simulink model "TeamA_PAsqualo_R19b"  (R2019b)
settings: Solver=VariableStepAuto  StartTime=0.0  StopTime=stop_time  FixedStep=0.05  RelTol=1e-3
InitFcn:
  | main_init
values from neighbouring files (symbols this model uses):
  a1 = rho * D^4 * alpha1    (= 0.000388302366464)    [data_current.m]    (also in main_init.m)
  a2 = -rho * D^3 * alpha2 * (1 - omega)    (= 0.0037030698432)    [data_current.m]    (also in main_init.m)
  ag = [Ax Ay Az]'    [init_modello.m]
  alpha1 = 0.0113    [data_current.m]    (also in main_init.m)
  alpha2 = -0.0091    [data_current.m]    (also in main_init.m)
  areaOfInterestCorner = [42.317744;10.915136; 0]    [init_controllo.m]    (also in missionA.m = [42.317744)
  bg = [Bx By Bz]'    [init_modello.m]
  cd_pitch = 0.7    [init_modello.m]
  cd_roll = 0.04    [init_modello.m]
  cd_x = 0.4    [init_modello.m]
  cd_y = 1    [init_modello.m]
  cd_yaw = 0.7    [init_modello.m]
  cd_z = 1    [init_modello.m]
  cg = [Cx Cy Cz]'    [init_modello.m]
  D = 0.076    [data_current.m]    (also in main_init.m)
  dead_zone_limit = 31.5    [data_current.m]    (also in main_init.m)
  dg = [Dx Dy Dz]'    [init_modello.m]
  eg = [Ex Ey Ez]'    [init_modello.m]
  fg = [Fx Fy Fz]'    [init_modello.m]
  g = 9.81    [init_modello.m]
  galleggiamento = 66.5386    [init_controllo.m]
  gg = [Gx Gy Gz]'    [init_modello.m]
  H0 = 0    [init_modello.m]
  init_position = [pointP(1),pointP(2),0.15,0,0,deg2rad(angle)]'    [appunti.m]    (also in init_modello.m = [pointP(1),pointP(2),0.15,0,0,deg2rad(alpha)]')
  init_velocity = [0 0 0 0 0 0]'    [init_modello.m]
  initial_state_cov = blkdiag(diag(cov_gps(1,1:2)), cov_depth*eye(n_state_filter-2))    [init_navigazione.m]
  Ixx = 0.93304097392    [init_modello.m]
  Ixy = 0    [init_modello.m]
  Ixz = 0    [init_modello.m]
  Iyy = 25.58745481378    (= 25.5874548138)    [init_modello.m]
  Iyz = 0    [init_modello.m]
  Izz = 25.58745481378    (= 25.5874548138)    [init_modello.m]
  K_i_heave_div = 20    [init_controllo.m]
  K_i_heave_pos = 1    [init_controllo.m]
  K_i_heave_surf = 20    [init_controllo.m]
  K_i_heave_trans = 5    [init_controllo.m]
  K_i_heave_turn = 5    [init_controllo.m]
  K_i_pitch_div = 0    [init_controllo.m]
  K_i_pitch_pos = 0.1*0    (= 0)    [init_controllo.m]
  K_i_pitch_surf = 0    [init_controllo.m]
  K_i_pitch_trans = 0    [init_controllo.m]
  K_i_pitch_turn = 0    [init_controllo.m]
  K_i_roll_div = 0    [init_controllo.m]
  K_i_roll_pos = 0.1*0    (= 0)    [init_controllo.m]
  K_i_roll_surf = 1    [init_controllo.m]
  K_i_roll_trans = 0    [init_controllo.m]
  K_i_roll_turn = 0    [init_controllo.m]
  K_i_surge_div = 3    [init_controllo.m]
  K_i_surge_pos = 0.1679*30    (= 5.037)    [init_controllo.m]
  K_i_surge_surf = 3    [init_controllo.m]
  K_i_surge_trans = 0.1679*15    (= 2.5185)    [init_controllo.m]
  K_i_surge_turn = 0.1679*60    (= 10.074)    [init_controllo.m]
  K_i_sway_div = 6    [init_controllo.m]
  K_i_sway_pos = 5    [init_controllo.m]
  K_i_sway_surf = 3    [init_controllo.m]
  K_i_sway_trans = 2    [init_controllo.m]
  K_i_sway_turn = 50    [init_controllo.m]
  K_i_yaw_div = 0    [init_controllo.m]
  K_i_yaw_pos = 1    [init_controllo.m]
  K_i_yaw_surf = 0    [init_controllo.m]
  K_i_yaw_trans = 20    [init_controllo.m]
  K_p_heave_div = 200    [init_controllo.m]
  K_p_heave_pos = 320    [init_controllo.m]
  K_p_heave_surf = 200    [init_controllo.m]
  K_p_heave_trans = 170    [init_controllo.m]
  K_p_heave_turn = 170    [init_controllo.m]
  K_p_phi_div = 0.15    [init_controllo.m]
  K_p_phi_pos = 1*0.1    (= 0.1)    [init_controllo.m]
  K_p_phi_surf = 0.15    [init_controllo.m]
  K_p_phi_trans = 0.1    [init_controllo.m]
  K_p_phi_turn = 0.1    [init_controllo.m]
  K_p_pitch_div = 50    [init_controllo.m]
  K_p_pitch_pos = 25    [init_controllo.m]
  K_p_pitch_surf = 50    [init_controllo.m]
  K_p_pitch_trans = 25    [init_controllo.m]
  K_p_pitch_turn = 25    [init_controllo.m]
  K_p_psi_div = 0.3    [init_controllo.m]
  K_p_psi_pos = 0.25    [init_controllo.m]
  K_p_psi_surf = 0.3    [init_controllo.m]
  K_p_psi_trans = 0.2    [init_controllo.m]
  K_p_roll_div = 10    [init_controllo.m]
  K_p_roll_pos = 0.1*40    (= 4)    [init_controllo.m]
  K_p_roll_surf = 10    [init_controllo.m]
  K_p_roll_trans = 0.1*40    (= 4)    [init_controllo.m]
  K_p_roll_turn = 4    [init_controllo.m]
  K_p_surge_div = 80    [init_controllo.m]
  K_p_surge_pos = 13.7782*2.5    (= 34.4455)    [init_controllo.m]
  K_p_surge_surf = 80    [init_controllo.m]
  K_p_surge_trans = 20    [init_controllo.m]
  K_p_surge_turn = 150    [init_controllo.m]
  K_p_sway_div = 100    [init_controllo.m]
  K_p_sway_pos = 90    [init_controllo.m]
  K_p_sway_surf = 80    [init_controllo.m]
  K_p_sway_trans = 80    [init_controllo.m]
  K_p_sway_turn = 200    [init_controllo.m]
  K_p_th_div = 0.3    [init_controllo.m]
  K_p_th_pos = 0.1    [init_controllo.m]
  K_p_th_surf = 0.3    [init_controllo.m]
  K_p_th_trans = 0.1    [init_controllo.m]
  K_p_th_turn = 0.1    [init_controllo.m]
  K_p_x_div = 0.12    [init_controllo.m]
  K_p_x_pos = 0.12    [init_controllo.m]
  K_p_x_surf = 0.12    [init_controllo.m]
  K_p_y_div = 0.6    [init_controllo.m]
  K_p_y_pos = 0.34    [init_controllo.m]
  K_p_y_surf = 0.1    [init_controllo.m]
  K_p_y_trans = 0.3    [init_controllo.m]
  K_p_y_turn = 0.3    [init_controllo.m]
  K_p_yaw_div = 70    [init_controllo.m]
  K_p_yaw_pos = 20    [init_controllo.m]
  K_p_yaw_surf = 70    [init_controllo.m]
  K_p_yaw_trans = 160    [init_controllo.m]
  K_p_z_div = 0.35    [init_controllo.m]
  K_p_z_pos = 0.2    [init_controllo.m]
  K_p_z_surf = 0.35    [init_controllo.m]
  K_p_z_trans = 0.10    (= 0.1)    [init_controllo.m]
  K_p_z_turn = 0.1    [init_controllo.m]
  Kadd = 0    [init_modello.m]
  m = 100    [init_modello.m]    (also in retta.m = p2-p1)
  Madd = -((((1/5)*(b^2-a^2)^2))*(alpha_0-beta_0))/((((2*(b^2-a^2)^2))+(b^2-a^2)^2)*(alpha_0-beta_0)*m)    [init_modello.m]
  ... (+59 more)
undefined symbols (not defined in the file or in its folder): DiscIntNeverNeededParam, initial_state
libraries: simulink x2, vrlib x1
(part 5 of 6)

== matlab function TeamA_PAsqualo_R19b/controller1/diving controller/heave_controller/Heave PID controller/compute_position_errors ==
  settings: updateMethod=DISCRETE  sampleTime=0.1
  data: enable input size=1; err_pos output size=1; ref input size=[12 1]; est_state input size=[12 1]; w_des output size=1; areaOfInterestCorner parameter
function [err_pos, w_des] = fcn(enable, ref, est_state,areaOfInterestCorner)
references_NED = zeros(3,1);
est_state_NED  = zeros(3,1);
phi = est_state(4);
th  = est_state(5);
psi = est_state(6);
coder.extrinsic('evalin','wgs84Ellipsoid','geodetic2ned');
orig = [areaOfInterestCorner(1)   areaOfInterestCorner(2)   areaOfInterestCorner(3)]'; %origine terna NED
wgs84 = wgs84Ellipsoid;
err_pos = 0;
w_des = 0;
if enable == 1
    % Cambiamento di riferimento da WGS84 a NED frame
   [x_ref, y_ref, z_ref] = geodetic2ned(ref(1),ref(2),ref(3),orig(1),orig(2),orig(3),wgs84);
   references_NED = [x_ref, y_ref, z_ref]';
   [x_est, y_est, z_est] = geodetic2ned(est_state(1),est_state(2),est_state(3),orig(1),orig(2),orig(3),wgs84);
   est_state_NED  =  [x_est, y_est, z_est]';
   est_state_NED = [est_state_NED(1);est_state_NED(2);est_state(3)];
   % Calcolo errore posizione da NED a BODY frame
   err_NED  = references_NED - est_state_NED;
   R_z_psi = [cos(psi)    sin(psi)     0;
              -sin(psi)   cos(psi)     0;
                 0           0         1];
          
   R_y_th =  [cos(th)        0      -sin(th);
                 0           1         0;
              sin(th)        0       cos(th)];
       
   R_x_phi = [   1           0             0;
                 0         cos(phi)    sin(phi);
                 0        -sin(phi)    cos(phi)];
          
   R_NB = ((R_z_psi')*(R_y_th')*(R_x_phi'))';
   err_pos_BODY = R_NB * err_NED;
   offset = 0.5;  % metri di distanza dal punto desiderato
   if err_pos_BODY(3) > offset
       err_pos = 0;
       w_des   = ref(9);
   end
   if err_pos_BODY(3) <= offset
       err_pos = err_pos_BODY(3);
       w_des   = 0;
   end
else
   err_pos = 0;
   w_des   = 0;
end
end

== matlab function TeamA_PAsqualo_R19b/controller1/diving controller/heave_controller/Heave PID controller/compute_velocity_error ==
  settings: updateMethod=DISCRETE  sampleTime=0.1
  data: enable input size=1; err_vel output size=1; v_des input size=1; est_meas input size=[12 1]
function err_vel = fcn(enable,v_des,est_meas)
if enable == 1
   err_vel =  v_des - est_meas(9);
else
    err_vel = 0;
end
end

== matlab function TeamA_PAsqualo_R19b/controller1/diving controller/pitch_controller/Pitch PID controller/compute_orientation_errors ==
  settings: updateMethod=DISCRETE  sampleTime=0.1
  data: enable input size=1; err_orient output size=1; ref input size=[12 1]; est_state input size=[12 1]
function err_orient = fcn(enable, ref, est_state)
coder.extrinsic('wrapToPi');
err_orient = 0;
phi = est_state(4);
th  = est_state(5);
%
J_inv = [1       0          -sin(th); 
         0   cos(phi)  cos(th)*sin(phi);
         0  -sin(phi)  cos(th)*cos(phi)];
if enable == 1
   err_orient_1 = wrapToPi(J_inv*([ref(4);ref(5);ref(6)] -...
                           [est_state(4);est_state(5);est_state(6)]));
else 
   err_orient_1 = zeros(3,1);
end
err_orient = err_orient_1(2);
end

== matlab function TeamA_PAsqualo_R19b/controller1/diving controller/pitch_controller/Pitch PID controller/compute_velocity_error ==
  settings: updateMethod=DISCRETE  sampleTime=0.1
  data: enable input size=1; err_vel output size=1; v_des input size=1; est_meas input size=[12 1]
function err_vel = fcn(enable,v_des,est_meas)
if enable == 1
   err_vel =  v_des - est_meas(11);
else
    err_vel = 0;
end
end

== matlab function TeamA_PAsqualo_R19b/controller1/diving controller/roll_controller/Roll PID controller/compute_orientation_errors ==
  settings: updateMethod=DISCRETE  sampleTime=0.1
  data: enable input size=1; err_orient output size=1; ref input size=[12 1]; est_state input size=[12 1]
function err_orient = fcn(enable, ref, est_state)
coder.extrinsic('wrapToPi');
err_orient = 0;
phi = est_state(4);
th  = est_state(5);
%
J_inv = [1       0          -sin(th); 
         0   cos(phi)  cos(th)*sin(phi);
         0  -sin(phi)  cos(th)*cos(phi)];
if enable == 1
   err_orient_1 = wrapToPi(J_inv*([ref(4);ref(5);ref(6)] -...
                           [est_state(4);est_state(5);est_state(6)]));
else 
   err_orient_1 = zeros(3,1);
end
err_orient = err_orient_1(1);
end

== matlab function TeamA_PAsqualo_R19b/controller1/diving controller/roll_controller/Roll PID controller/compute_velocity_error ==
  settings: updateMethod=DISCRETE  sampleTime=0.1
  data: enable input size=1; err_vel output size=1; v_des input size=1; est_meas input size=[12 1]
function err_vel = fcn(enable,v_des,est_meas)
if enable == 1
   err_vel =  v_des - est_meas(10);
else
    err_vel = 0;
end
end

== matlab function TeamA_PAsqualo_R19b/controller1/diving controller/surge_controller/Surge PID controller/compute_position_errors ==
  settings: updateMethod=DISCRETE  sampleTime=0.1
  data: enable input size=1; err_pos output size=1; ref input size=[12 1]; est_state input size=[12 1]; areaOfInterestCorner parameter
function err_pos = fcn(enable, ref, est_state,areaOfInterestCorner)
references_NED = zeros(3,1);
est_state_NED  = zeros(3,1);
phi = est_state(4);
th  = est_state(5);
psi = est_state(6);
coder.extrinsic('evalin','wgs84Ellipsoid','geodetic2ned');
orig = [areaOfInterestCorner(1)   areaOfInterestCorner(2)   areaOfInterestCorner(3)]'; %origine terna NED
wgs84 = wgs84Ellipsoid;
if enable == 1
    % Cambiamento di riferimento da WGS84 a NED frame
   [x_ref, y_ref, z_ref] = geodetic2ned(ref(1),ref(2),ref(3),orig(1),orig(2),orig(3),wgs84);
   references_NED = [x_ref, y_ref, z_ref]';
   [x_est, y_est, z_est] = geodetic2ned(est_state(1),est_state(2),est_state(3),orig(1),orig(2),orig(3),wgs84);
   est_state_NED  =  [x_est, y_est, est_state(3)]';
   % Calcolo errore posizione da NED a BODY frame
   err_NED  = references_NED - est_state_NED;
   R_z_psi = [cos(psi)    sin(psi)     0;
              -sin(psi)   cos(psi)     0;
                 0           0         1];
          
   R_y_th =  [cos(th)        0      -sin(th);
                 0           1         0;
              sin(th)        0       cos(th)];
       
   R_x_phi = [   1           0             0;
                 0         cos(phi)    sin(phi);
                 0        -sin(phi)    cos(phi)];
          
   R_NB = ((R_z_psi')*(R_y_th')*(R_x_phi'))';
   err_pos_BODY = R_NB * err_NED;

   err_pos = err_pos_BODY(1);
else
   err_pos = 0;
end
end

== matlab function TeamA_PAsqualo_R19b/controller1/diving controller/surge_controller/Surge PID controller/compute_velocity_error ==
  settings: updateMethod=DISCRETE  sampleTime=0.1
  data: enable input size=1; err_vel output size=1; v_des input size=1; est_meas input size=[12 1]
function err_vel = fcn(enable,v_des,est_meas)
if enable == 1
   err_vel =  v_des - est_meas(7);
else
    err_vel = 0;
end
end

== matlab function TeamA_PAsqualo_R19b/controller1/diving controller/sway_controller/Sway PID controller/compute_position_errors ==
  settings: updateMethod=DISCRETE  sampleTime=0.1
  data: enable input size=1; err_pos output size=1; ref input size=[12 1]; est_state input size=[12 1]; areaOfInterestCorner parameter
function err_pos = fcn(enable, ref, est_state,areaOfInterestCorner)
references_NED = zeros(3,1);
est_state_NED  = zeros(3,1);
phi = est_state(4);
th  = est_state(5);
psi = est_state(6);
coder.extrinsic('evalin','wgs84Ellipsoid','geodetic2ned');
orig = [areaOfInterestCorner(1)   areaOfInterestCorner(2)   areaOfInterestCorner(3)]'; %origine terna NED
wgs84 = wgs84Ellipsoid;
if enable == 1
    % Cambiamento di riferimento da WGS84 a NED frame
   [x_ref, y_ref, z_ref] = geodetic2ned(ref(1),ref(2),ref(3),orig(1),orig(2),orig(3),wgs84);
   references_NED = [x_ref, y_ref, z_ref]';
   [x_est, y_est, z_est] = geodetic2ned(est_state(1),est_state(2),est_state(3),orig(1),orig(2),orig(3),wgs84);
   est_state_NED  = [x_est, y_est, est_state(3)]';
   % Calcolo errore posizione da NED a BODY frame
   err_NED  = references_NED - est_state_NED;
   R_z_psi = [cos(psi)    sin(psi)     0;
              -sin(psi)   cos(psi)     0;
                 0           0         1];
          
   R_y_th =  [cos(th)        0      -sin(th);
                 0           1         0;
              sin(th)        0       cos(th)];
       
   R_x_phi = [   1           0             0;
                 0         cos(phi)    sin(phi);
                 0        -sin(phi)    cos(phi)];
          
   R_NB = ((R_z_psi')*(R_y_th')*(R_x_phi'))';
   err_pos_BODY = R_NB * err_NED;
   err_pos = err_pos_BODY(2);
else
   err_pos = 0;
end
end

== matlab function TeamA_PAsqualo_R19b/controller1/diving controller/sway_controller/Sway PID controller/compute_velocity_error ==
  settings: updateMethod=DISCRETE  sampleTime=0.1
  data: enable input size=1; err_vel output size=1; v_des input size=1; est_meas input size=[12 1]
function err_vel = fcn(enable,v_des,est_meas)
if enable == 1
   err_vel =  v_des - est_meas(8);
else
    err_vel = 0;
end
end

== matlab function TeamA_PAsqualo_R19b/controller1/diving controller/yaw_controller/Yaw PID controller/compute_orientation_errors ==
  settings: updateMethod=DISCRETE  sampleTime=0.1
  data: enable input size=1; err_orient output size=1; ref input size=[12 1]; est_state input size=[12 1]
function err_orient = fcn(enable, ref, est_state)
coder.extrinsic('wrapToPi');
err_orient = 0;
phi = est_state(4);
th  = est_state(5);
%
J_inv = [1       0          -sin(th); 
         0   cos(phi)  cos(th)*sin(phi);
         0  -sin(phi)  cos(th)*cos(phi)];
if enable == 1
   err_orient_1 = wrapToPi(J_inv*([ref(4);ref(5);ref(6)] -...
                           [est_state(4);est_state(5);est_state(6)]));
else 
   err_orient_1 = zeros(3,1);
end
err_orient = err_orient_1(3);
end

== matlab function TeamA_PAsqualo_R19b/controller1/diving controller/yaw_controller/Yaw PID controller/compute_velocity_error ==
  data: enable input; err_vel output; v_des input; est_meas input
function err_vel = fcn(enable,v_des,est_meas)
if enable == 1
   err_vel =  v_des - est_meas(12);
else
    err_vel = 0;
end

== matlab function TeamA_PAsqualo_R19b/controller1/positioning controller/heave_controller/Heave PID controller/compute_position_errors ==
  data: enable input; err_pos output; ref input; est_state input; areaOfInterestCorner parameter
function err_pos = fcn(enable, ref, est_state,areaOfInterestCorner)
references_NED = zeros(3,1);
est_state_NED  = zeros(3,1);
phi = est_state(4);
th  = est_state(5);
psi = est_state(6);
coder.extrinsic('evalin','wgs84Ellipsoid','geodetic2ned');   
orig = [areaOfInterestCorner(1)   areaOfInterestCorner(2)   areaOfInterestCorner(3)]'; %origine terna NED
wgs84 = wgs84Ellipsoid;
if enable == 1
    % Cambiamento di riferimento da WGS84 a NED frame
   [x_ref, y_ref, z_ref] = geodetic2ned(ref(1),ref(2),ref(3),orig(1),orig(2),orig(3),wgs84);
   references_NED = [x_ref, y_ref, z_ref]';
   [x_est, y_est, z_est] = geodetic2ned(est_state(1),est_state(2),est_state(3),orig(1),orig(2),orig(3),wgs84);
   est_state_NED  =  [x_est, y_est, est_state(3)]';
   % Calcolo errore posizione da NED a BODY frame
   err_NED  = references_NED - est_state_NED;
   R_z_psi = [cos(psi)    sin(psi)     0;
              -sin(psi)   cos(psi)     0;
                 0           0         1];
          
   R_y_th =  [cos(th)        0      -sin(th);
                 0           1         0;
              sin(th)        0       cos(th)];
       
   R_x_phi = [   1           0             0;
                 0         cos(phi)    sin(phi);
                 0        -sin(phi)    cos(phi)];
          
   R_NB = ((R_z_psi')*(R_y_th')*(R_x_phi'))';
   err_pos_BODY = R_NB * err_NED;
   err_pos = err_pos_BODY(3);
else
   err_pos = 0;
end
end

== matlab function TeamA_PAsqualo_R19b/controller1/positioning controller/heave_controller/Heave PID controller/compute_velocity_error ==
  data: enable input; err_vel output; v_des input; est_meas input
function err_vel = fcn(enable,v_des,est_meas)
err_vel = 0;
if enable == 1
   err_vel =  v_des - est_meas(9);
else 
    err_vel = 0;
end
end

== matlab function TeamA_PAsqualo_R19b/controller1/positioning controller/pitch_controller/Pitch PID controller/compute_orientation_errors ==
  data: enable input; err_orient output; ref input; est_state input
function err_orient = fcn(enable, ref, est_state)
coder.extrinsic('wrapToPi');
err_orient = 0;
phi = est_state(4);
th  = est_state(5);
%
J_inv = [1       0          -sin(th); 
         0   cos(phi)  cos(th)*sin(phi);
         0  -sin(phi)  cos(th)*cos(phi)];
if enable == 1
   err_orient_1 = wrapToPi(J_inv*([ref(4);ref(5);ref(6)] -...
                                [est_state(4);est_state(5);est_state(6)]));
else 
   err_orient_1 = zeros(3,1);
end
err_orient = err_orient_1(2);
end

== matlab function TeamA_PAsqualo_R19b/controller1/positioning controller/pitch_controller/Pitch PID controller/compute_velocity_error ==
  data: enable input; err_vel output; v_des input; est_meas input
function err_vel = fcn(enable,v_des,est_meas)
if enable == 1
   err_vel =  v_des - est_meas(11);
else
    err_vel = 0;
end
end

== matlab function TeamA_PAsqualo_R19b/controller1/positioning controller/roll_controller/Roll PID controller/compute_orientation_errors ==
  data: enable input; err_orient output; ref input; est_state input
function err_orient = fcn(enable, ref, est_state)
coder.extrinsic('wrapToPi');
err_orient = 0;
phi = est_state(4);
th  = est_state(5);
%
J_inv = [1       0          -sin(th); 
         0   cos(phi)  cos(th)*sin(phi);
         0  -sin(phi)  cos(th)*cos(phi)];
if enable == 1
   err_orient_1 = wrapToPi(J_inv*([ref(4);ref(5);ref(6)] -...
                           [est_state(4);est_state(5);est_state(6)]));
else 
   err_orient_1 = zeros(3,1);
end
err_orient = err_orient_1(1);
end

== matlab function TeamA_PAsqualo_R19b/controller1/positioning controller/roll_controller/Roll PID controller/compute_velocity_error ==
  data: enable input; err_vel output; v_des input; est_meas input
function err_vel = fcn(enable,v_des,est_meas)
if enable == 1
   err_vel =  v_des - est_meas(10);
else 
    err_vel = 0;
end
end

== matlab function TeamA_PAsqualo_R19b/controller1/positioning controller/surge_controller/Surge PID controller/compute_position_errors ==
  data: enable input; err_pos output; ref input; est_state input; u_des output; areaOfInterestCorner parameter
function [err_pos, u_des] = fcn(enable, ref, est_state,areaOfInterestCorner)
references_NED = zeros(3,1);
est_state_NED  = zeros(3,1);
phi = est_state(4);
th  = est_state(5);
psi = est_state(6);
coder.extrinsic('evalin','wgs84Ellipsoid','geodetic2ned');
orig = [areaOfInterestCorner(1)   areaOfInterestCorner(2)   areaOfInterestCorner(3)]'; %origine terna NED
wgs84 = wgs84Ellipsoid;
err_pos = 0;
u_des = 0;

if enable == 1
    % Cambiamento di riferimento da WGS84 a NED frame
   [x_ref, y_ref, z_ref] = geodetic2ned(ref(1),ref(2),ref(3),orig(1),orig(2),orig(3),wgs84);
   references_NED = [x_ref, y_ref, z_ref]';
   [x_est, y_est, z_est] = geodetic2ned(est_state(1),est_state(2),est_state(3),orig(1),orig(2),orig(3),wgs84);
   est_state_NED  =  [x_est, y_est, z_est]';
   est_state_NED = [est_state_NED(1);est_state_NED(2);est_state(3)];
   % Calcolo errore posizione da NED a BODY frame
   err_NED  = references_NED - est_state_NED;
   R_z_psi = [cos(psi)    sin(psi)     0;
              -sin(psi)   cos(psi)     0;
                 0           0         1];
          
   R_y_th =  [cos(th)        0      -sin(th);
                 0           1         0;
              sin(th)        0       cos(th)];
       
   R_x_phi = [   1           0             0;
                 0         cos(phi)    sin(phi);
                 0        -sin(phi)    cos(phi)];
          
   R_NB = ((R_z_psi')*(R_y_th')*(R_x_phi'))';
   err_pos_BODY = R_NB * err_NED;
   offset = 5;  % metri di distanza dal punto desiderato
   if abs(err_pos_BODY(1)) > offset
       err_pos = 0;
       u_des   = ref(7);
   end
   if abs(err_pos_BODY(1)) <= offset
       err_pos = err_pos_BODY(1);
       u_des   = 0;
   end
else
   err_pos = 0;
   u_des   = 0;
end
end

== matlab function TeamA_PAsqualo_R19b/controller1/positioning controller/surge_controller/Surge PID controller/compute_velocity_error ==
  data: enable input; err_vel output; v_des input; est_meas input
function err_vel = fcn(enable,v_des,est_meas)
if enable == 1
   err_vel =  v_des - est_meas(7);
else
    err_vel = 0;
end
end

== matlab function TeamA_PAsqualo_R19b/controller1/positioning controller/sway_controller/Sway PID controller/compute_position_errors ==
  data: enable input; err_pos output; ref input; est_state input; areaOfInterestCorner parameter
function err_pos = fcn(enable, ref, est_state,areaOfInterestCorner)
references_NED = zeros(3,1);
est_state_NED  = zeros(3,1);
phi = est_state(4);
th  = est_state(5);
psi = est_state(6);
coder.extrinsic('evalin','wgs84Ellipsoid','geodetic2ned');   
orig = [areaOfInterestCorner(1)   areaOfInterestCorner(2)   areaOfInterestCorner(3)]'; %origine terna NED
wgs84 = wgs84Ellipsoid;
if enable == 1
    % Cambiamento di riferimento da WGS84 a NED frame
   [x_ref, y_ref, z_ref] = geodetic2ned(ref(1),ref(2),ref(3),orig(1),orig(2),orig(3),wgs84);
   references_NED = [x_ref, y_ref, z_ref]';
   [x_est, y_est, z_est] = geodetic2ned(est_state(1),est_state(2),est_state(3),orig(1),orig(2),orig(3),wgs84);
   est_state_NED  =  [x_est, y_est, est_state(3)]';
   % Calcolo errore posizione da NED a BODY frame
   err_NED  = references_NED - est_state_NED;
   %
   R_z_psi = [cos(psi)    sin(psi)     0;
              -sin(psi)   cos(psi)     0;
                 0           0         1];
          
   R_y_th =  [cos(th)        0      -sin(th);
                 0           1         0;
              sin(th)        0       cos(th)];
       
   R_x_phi = [   1           0             0;
                 0         cos(phi)    sin(phi);
                 0        -sin(phi)    cos(phi)];
          
   R_NB = ((R_z_psi')*(R_y_th')*(R_x_phi'))'; % matrice rotazione NED->BODY
   err_pos_BODY = R_NB * err_NED;
   err_pos = err_pos_BODY(2);
else 
   err_pos = 0;
end
end

== matlab function TeamA_PAsqualo_R19b/controller1/positioning controller/sway_controller/Sway PID controller/compute_velocity_error ==
  data: enable input; err_vel output; v_des input; est_meas input
function err_vel = fcn(enable,v_des,est_meas)
if enable == 1
   err_vel =  v_des - est_meas(8);

else 
    err_vel = 0;
end
end

== matlab function TeamA_PAsqualo_R19b/controller1/positioning controller/yaw_controller/Yaw PID controller/compute_orientation_errors ==
  data: enable input; err_orient output; ref input; est_state input
function err_orient = fcn(enable, ref, est_state)
coder.extrinsic('wrapToPi');
err_orient = 0;
phi = est_state(4);
th  = est_state(5);
%
J_inv = [1       0          -sin(th); 
         0   cos(phi)  cos(th)*sin(phi);
         0  -sin(phi)  cos(th)*cos(phi)];
if enable == 1
   err_orient_1 = wrapToPi(J_inv*([ref(4);ref(5);ref(6)] -...
                           [est_state(4);est_state(5);est_state(6)]));
else 
   err_orient_1 = zeros(3,1);
end
err_orient = err_orient_1(3);
end

== matlab function TeamA_PAsqualo_R19b/controller1/positioning controller/yaw_controller/Yaw PID controller/compute_velocity_error ==
  data: enable input; err_vel output; v_des input; est_meas input
function err_vel = fcn(enable,v_des,est_meas)
if enable == 1
   err_vel =  v_des - est_meas(12);
else
    err_vel = 0;
end
end

== matlab function TeamA_PAsqualo_R19b/controller1/surfacing controller/heave_controller/Heave PID controller/compute_position_errors ==
  data: enable input; err_pos output; ref input; est_state input; w_des output; areaOfInterestCorner parameter
function [err_pos, w_des] = fcn(enable, ref, est_state,areaOfInterestCorner)
references_NED = zeros(3,1);
est_state_NED  = zeros(3,1);
phi = est_state(4);
th  = est_state(5);
psi = est_state(6);
coder.extrinsic('evalin','wgs84Ellipsoid','geodetic2ned');
orig = [areaOfInterestCorner(1)   areaOfInterestCorner(2)   areaOfInterestCorner(3)]'; %origine terna NED
wgs84 = wgs84Ellipsoid;
err_pos = 0;
w_des = 0;
if enable == 1
    % Cambiamento di riferimento da WGS84 a NED frame
   [x_ref, y_ref, z_ref] = geodetic2ned(ref(1),ref(2),ref(3),orig(1),orig(2),orig(3),wgs84);
   references_NED = [x_ref, y_ref, z_ref]';
   [x_est, y_est, z_est] = geodetic2ned(est_state(1),est_state(2),est_state(3),orig(1),orig(2),orig(3),wgs84);
   est_state_NED  =  [x_est, y_est, z_est]';
   est_state_NED = [est_state_NED(1);est_state_NED(2);est_state(3)];
   % Calcolo errore posizione da NED a BODY frame
   err_NED  = references_NED - est_state_NED;
   R_z_psi = [cos(psi)    sin(psi)     0;
              -sin(psi)   cos(psi)     0;
                 0           0         1];
          
   R_y_th =  [cos(th)        0      -sin(th);
                 0           1         0;
              sin(th)        0       cos(th)];
       
   R_x_phi = [   1           0             0;
                 0         cos(phi)    sin(phi);
                 0        -sin(phi)    cos(phi)];
          
   R_NB = ((R_z_psi')*(R_y_th')*(R_x_phi'))';
   err_pos_BODY = R_NB * err_NED;
   offset = -0.5;  % metri di distanza dal punto desiderato
   if err_pos_BODY(3) < offset
       err_pos = 0;
       w_des   = ref(9);
   end
   if err_pos_BODY(3) > offset
       err_pos = err_pos_BODY(3);
       w_des   = 0;
   end
else
   err_pos = 0;
   w_des   = 0;
end
end

== matlab function TeamA_PAsqualo_R19b/controller1/surfacing controller/heave_controller/Heave PID controller/compute_velocity_error ==
  data: enable input; err_vel output; v_des input; est_meas input
function err_vel = fcn(enable,v_des,est_meas)
if enable == 1
   err_vel =  v_des - est_meas(9);
else
    err_vel = 0;
end
end

== matlab function TeamA_PAsqualo_R19b/controller1/surfacing controller/pitch_controller/Pitch PID controller/compute_orientation_errors ==
  data: enable input; err_orient output; ref input; est_state input
function err_orient = fcn(enable, ref, est_state)
coder.extrinsic('wrapToPi');
err_orient = 0;
phi = est_state(4);
th  = est_state(5);
%
J_inv = [1       0          -sin(th); 
         0   cos(phi)  cos(th)*sin(phi);
         0  -sin(phi)  cos(th)*cos(phi)];
if enable == 1
   err_orient_1 = wrapToPi(J_inv*([ref(4);ref(5);ref(6)] -...
                           [est_state(4);est_state(5);est_state(6)]));
else 
   err_orient_1 = zeros(3,1);
end
err_orient = err_orient_1(2);
end

== matlab function TeamA_PAsqualo_R19b/controller1/surfacing controller/pitch_controller/Pitch PID controller/compute_velocity_error ==
  data: enable input; err_vel output; v_des input; est_meas input
function err_vel = fcn(enable,v_des,est_meas)
if enable == 1
   err_vel =  v_des - est_meas(11);
else
    err_vel = 0;
end
end

== matlab function TeamA_PAsqualo_R19b/controller1/surfacing controller/roll_controller/Roll PID controller/compute_orientation_errors ==
  data: enable input; err_orient output; ref input; est_state input
function err_orient = fcn(enable, ref, est_state)
coder.extrinsic('wrapToPi');
err_orient = 0;
phi = est_state(4);
th  = est_state(5);
%
J_inv = [1       0          -sin(th); 
         0   cos(phi)  cos(th)*sin(phi);
         0  -sin(phi)  cos(th)*cos(phi)];
if enable == 1
   err_orient_1 = wrapToPi(J_inv*([ref(4);ref(5);ref(6)] -...
                           [est_state(4);est_state(5);est_state(6)]));
else 
   err_orient_1 = zeros(3,1);
end
err_orient = err_orient_1(1);
end

== matlab function TeamA_PAsqualo_R19b/controller1/surfacing controller/roll_controller/Roll PID controller/compute_velocity_error ==
  data: enable input; err_vel output; v_des input; est_meas input
function err_vel = fcn(enable,v_des,est_meas)
if enable == 1
   err_vel =  v_des - est_meas(10);
else
    err_vel = 0;
end
end

== matlab function TeamA_PAsqualo_R19b/controller1/surfacing controller/surge_controller/Surge PID controller/compute_position_errors ==
  data: enable input; err_pos output; ref input; est_state input; areaOfInterestCorner parameter
function err_pos = fcn(enable, ref, est_state,areaOfInterestCorner)
references_NED = zeros(3,1);
est_state_NED  = zeros(3,1);
phi = est_state(4);
th  = est_state(5);
psi = est_state(6);
coder.extrinsic('evalin','wgs84Ellipsoid','geodetic2ned');
orig = [areaOfInterestCorner(1)   areaOfInterestCorner(2)   areaOfInterestCorner(3)]'; %origine terna NED
wgs84 = wgs84Ellipsoid;
if enable == 1
    % Cambiamento di riferimento da WGS84 a NED frame
   [x_ref, y_ref, z_ref] = geodetic2ned(ref(1),ref(2),ref(3),orig(1),orig(2),orig(3),wgs84);
   references_NED = [x_ref, y_ref, z_ref]';
   [x_est, y_est, z_est] = geodetic2ned(est_state(1),est_state(2),est_state(3),orig(1),orig(2),orig(3),wgs84);
   est_state_NED  =  [x_est, y_est, est_state(3)]';
   % Calcolo errore posizione da NED a BODY frame
   err_NED  = references_NED - est_state_NED;
   R_z_psi = [cos(psi)    sin(psi)     0;
              -sin(psi)   cos(psi)     0;
                 0           0         1];
          
   R_y_th =  [cos(th)        0      -sin(th);
                 0           1         0;
              sin(th)        0       cos(th)];
       
   R_x_phi = [   1           0             0;
                 0         cos(phi)    sin(phi);
                 0        -sin(phi)    cos(phi)];
          
   R_NB = ((R_z_psi')*(R_y_th')*(R_x_phi'))';
   err_pos_BODY = R_NB * err_NED;
   err_pos = err_pos_BODY(1);
else
   err_pos = 0;
end
end

== matlab function TeamA_PAsqualo_R19b/controller1/surfacing controller/surge_controller/Surge PID controller/compute_velocity_error ==
  data: enable input; err_vel output; v_des input; est_meas input
function err_vel = fcn(enable,v_des,est_meas)
if enable == 1
   err_vel =  v_des - est_meas(7);
else
    err_vel = 0;
end
end

== matlab function TeamA_PAsqualo_R19b/controller1/surfacing controller/sway_controller/Sway PID controller/compute_position_errors ==
  data: enable input; err_pos output; ref input; est_state input; areaOfInterestCorner parameter
function err_pos = fcn(enable, ref, est_state,areaOfInterestCorner)
references_NED = zeros(3,1);
est_state_NED  = zeros(3,1);
phi = est_state(4);
th  = est_state(5);
psi = est_state(6);
coder.extrinsic('evalin','wgs84Ellipsoid','geodetic2ned');
orig = [areaOfInterestCorner(1)   areaOfInterestCorner(2)   areaOfInterestCorner(3)]'; %origine terna NED
wgs84 = wgs84Ellipsoid;
if enable == 1
    % Cambiamento di riferimento da WGS84 a NED frame
   [x_ref, y_ref, z_ref] = geodetic2ned(ref(1),ref(2),ref(3),orig(1),orig(2),orig(3),wgs84);
   references_NED = [x_ref, y_ref, z_ref]';
   [x_est, y_est, z_est] = geodetic2ned(est_state(1),est_state(2),est_state(3),orig(1),orig(2),orig(3),wgs84);
   est_state_NED  =  [x_est, y_est,est_state(3)]';
   % Calcolo errore posizione da NED a BODY frame
   err_NED  = references_NED - est_state_NED;
   R_z_psi = [cos(psi)    sin(psi)     0;
              -sin(psi)   cos(psi)     0;
                 0           0         1];
          
   R_y_th =  [cos(th)        0      -sin(th);
                 0           1         0;
              sin(th)        0       cos(th)];
       
   R_x_phi = [   1           0             0;
                 0         cos(phi)    sin(phi);
                 0        -sin(phi)    cos(phi)];
          
   R_NB = ((R_z_psi')*(R_y_th')*(R_x_phi'))';
   err_pos_BODY = R_NB * err_NED;
   err_pos = err_pos_BODY(2);
else
   err_pos = 0;
end
end

== matlab function TeamA_PAsqualo_R19b/controller1/surfacing controller/sway_controller/Sway PID controller/compute_velocity_error ==
  data: enable input; err_vel output; v_des input; est_meas input
function err_vel = fcn(enable,v_des,est_meas)
if enable == 1
   err_vel =  v_des - est_meas(8);
else
    err_vel = 0;
end
end

== matlab function TeamA_PAsqualo_R19b/controller1/surfacing controller/yaw_controller/Yaw PID controller/compute_orientation_errors ==
  data: enable input; err_orient output; ref input; est_state input
function err_orient = fcn(enable, ref, est_state)
coder.extrinsic('wrapToPi');
err_orient = 0;
phi = est_state(4);
th  = est_state(5);
%
J_inv = [1       0          -sin(th); 
         0   cos(phi)  cos(th)*sin(phi);
         0  -sin(phi)  cos(th)*cos(phi)];
if enable == 1
   err_orient_1 = wrapToPi(J_inv*([ref(4);ref(5);ref(6)] -...
                           [est_state(4);est_state(5);est_state(6)]));
else 
   err_orient_1 = zeros(3,1);
end
err_orient = err_orient_1(3);
end

== matlab function TeamA_PAsqualo_R19b/controller1/surfacing controller/yaw_controller/Yaw PID controller/compute_velocity_error ==
  data: enable input; err_vel output; v_des input; est_meas input
function err_vel = fcn(enable,v_des,est_meas)
if enable == 1
   err_vel =  v_des - est_meas(12);
else
    err_vel = 0;
end
end

== matlab function TeamA_PAsqualo_R19b/controller1/transect controller/heave_controller/Heave PID controller/compute_position_errors ==
  data: enable input; err_pos output; ref input; est_state input; areaOfInterestCorner parameter
function err_pos = fcn(enable, ref, est_state,areaOfInterestCorner)
references_NED = zeros(3,1);
est_state_NED  = zeros(3,1);
phi = est_state(4);
th  = est_state(5);
psi = est_state(6);
coder.extrinsic('evalin','wgs84Ellipsoid','geodetic2ned');
orig = [areaOfInterestCorner(1)   areaOfInterestCorner(2)   areaOfInterestCorner(3)]'; %origine terna NED
wgs84 = wgs84Ellipsoid;
if enable == 1
    % Cambiamento di riferimento da WGS84 a NED frame
   [x_ref, y_ref, z_ref] = geodetic2ned(ref(1),ref(2),ref(3),orig(1),orig(2),orig(3),wgs84);
   references_NED = [x_ref, y_ref, z_ref]';
   [x_est, y_est, z_est] = geodetic2ned(est_state(1),est_state(2),est_state(3),orig(1),orig(2),orig(3),wgs84);
   est_state_NED  =  [x_est, y_est, z_est]';
   est_state_NED = [est_state_NED(1);est_state_NED(2);est_state(3)];
   % Calcolo errore posizione da NED a BODY frame
   err_NED  = references_NED - est_state_NED;
   R_z_psi = [cos(psi)    sin(psi)     0;
              -sin(psi)   cos(psi)     0;
                 0           0         1];
          
   R_y_th =  [cos(th)        0      -sin(th);
                 0           1         0;
              sin(th)        0       cos(th)];
       
   R_x_phi = [   1           0             0;
                 0         cos(phi)    sin(phi);
                 0        -sin(phi)    cos(phi)];
          
   R_NB = ((R_z_psi')*(R_y_th')*(R_x_phi'))';
   err_pos_BODY = R_NB * err_NED;
   err_pos = err_pos_BODY(3);
else
   err_pos = 0;
end
end

== matlab function TeamA_PAsqualo_R19b/controller1/transect controller/heave_controller/Heave PID controller/compute_velocity_error ==
  data: enable input; err_vel output; v_des input; est_meas input
function err_vel = fcn(enable,v_des,est_meas)
if enable == 1
   err_vel =  v_des - est_meas(9);
else
    err_vel = 0;
end
end

== matlab function TeamA_PAsqualo_R19b/controller1/transect controller/pitch_controller/Pitch PID controller/compute_orientation_errors ==
  data: enable input; err_orient output; ref input; est_state input
function err_orient = fcn(enable, ref, est_state)
coder.extrinsic('wrapToPi');
err_orient = 0;
phi = est_state(4);
th  = est_state(5);
%
J_inv = [1       0          -sin(th); 
         0   cos(phi)  cos(th)*sin(phi);
         0  -sin(phi)  cos(th)*cos(phi)];
if enable == 1
   err_orient_1 = wrapToPi(J_inv*([ref(4);ref(5);ref(6)] -...
                           [est_state(4);est_state(5);est_state(6)]));
else 
   err_orient_1 = zeros(3,1);
end
err_orient = err_orient_1(2);
end

== matlab function TeamA_PAsqualo_R19b/controller1/transect controller/pitch_controller/Pitch PID controller/compute_velocity_error ==
  data: enable input; err_vel output; v_des input; est_meas input
function err_vel = fcn(enable,v_des,est_meas)
if enable == 1
   err_vel =  v_des - est_meas(11);
else
    err_vel = 0;
end
end

== matlab function TeamA_PAsqualo_R19b/controller1/transect controller/roll_controller/Roll PID controller/compute_orientation_errors ==
  data: enable input; err_orient output; ref input; est_state input
function err_orient = fcn(enable, ref, est_state)
coder.extrinsic('wrapToPi');
err_orient = 0;
phi = est_state(4);
th  = est_state(5);
%
J_inv = [1       0          -sin(th); 
         0   cos(phi)  cos(th)*sin(phi);
         0  -sin(phi)  cos(th)*cos(phi)];
if enable == 1
   err_orient_1 = wrapToPi(J_inv*([ref(4);ref(5);ref(6)] -...
                           [est_state(4);est_state(5);est_state(6)]));
else 
   err_orient_1 = zeros(3,1);
end
err_orient = err_orient_1(1);
end

== matlab function TeamA_PAsqualo_R19b/controller1/transect controller/roll_controller/Roll PID controller/compute_velocity_error ==
  data: enable input; err_vel output; v_des input; est_meas input
function err_vel = fcn(enable,v_des,est_meas)
if enable == 1
   err_vel =  v_des - est_meas(10);
else
    err_vel = 0;
end
end

== matlab function TeamA_PAsqualo_R19b/controller1/transect controller/surge_controller/Surge PID controller/ compute_velocity_error ==
  data: enable input; ref input; est_meas input; err_vel output
function err_vel = fcn(enable, ref, est_meas)
if  enable == 1
    err_vel = ref(7) - est_meas(7);
else
    err_vel = 0;
end
end

== matlab function TeamA_PAsqualo_R19b/controller1/transect controller/sway_controller/Sway PID controller/compute_position_errors ==
  data: enable input; err_pos output; ref input; est_state input; areaOfInterestCorner parameter
function err_pos = fcn(enable, ref, est_state,areaOfInterestCorner)
coder.extrinsic('wrapToPi');
coder.extrinsic('evalin','wgs84Ellipsoid','geodetic2ned');
references_NED = zeros(3,1);
est_state_NED  = zeros(3,1);
phi = est_state(4);
th  = est_state(5);
psi = est_state(6);
psi = wrapToPi(psi);
orig = [areaOfInterestCorner(1)   areaOfInterestCorner(2)   areaOfInterestCorner(3)]'; %origine terna NED
wgs84 = wgs84Ellipsoid;
if enable == 1
    % Cambiamento di riferimento da WGS84 a NED frame
   [x_ref, y_ref, z_ref] = geodetic2ned(ref(1),ref(2),ref(3),orig(1),orig(2),orig(3),wgs84);
   references_NED = [x_ref, y_ref, z_ref]';
   [x_est, y_est, z_est] = geodetic2ned(est_state(1),est_state(2),est_state(3),orig(1),orig(2),orig(3),wgs84);
   est_state_NED  =  [x_est, y_est, est_state(3)]';
   % Calcolo errore posizione da NED a BODY frame
   err_NED  = references_NED - est_state_NED;
   R_z_psi = [cos(psi)    sin(psi)     0;
              -sin(psi)   cos(psi)     0;
                 0           0         1];
          
   R_y_th =  [cos(th)        0      -sin(th);
                 0           1         0;
              sin(th)        0       cos(th)];
       
   R_x_phi = [   1           0             0;
                 0         cos(phi)    sin(phi);
                 0        -sin(phi)    cos(phi)];
          
   R_NB = ((R_z_psi')*(R_y_th')*(R_x_phi'))';
   err_pos_BODY = R_NB * err_NED;
   err_pos = err_pos_BODY(2);
else
   err_pos = 0;
end
end

== matlab function TeamA_PAsqualo_R19b/controller1/transect controller/sway_controller/Sway PID controller/compute_velocity_error ==
  data: enable input; err_vel output; v_des input; est_meas input
function err_vel = fcn(enable,v_des,est_meas)
if enable == 1
   err_vel =  v_des - est_meas(8);
else
    err_vel = 0;
end
end

== matlab function TeamA_PAsqualo_R19b/controller1/transect controller/yaw_controller/Yaw PID controller/compute_orientation_errors ==
  data: enable input; err_orient output; ref input; est_state input
function err_orient = fcn(enable, ref, est_state)
coder.extrinsic('wrapToPi');
err_orient = 0;
phi = est_state(4);
th  = est_state(5);
%
J_inv = [1       0          -sin(th); 
         0   cos(phi)  cos(th)*sin(phi);
         0  -sin(phi)  cos(th)*cos(phi)];
if enable == 1
   err_orient_1 = wrapToPi(J_inv*([ref(4);ref(5);ref(6)] -...
                           [est_state(4);est_state(5);est_state(6)]));
else 
   err_orient_1 = zeros(3,1);
end
err_orient = err_orient_1(3);
end

== matlab function TeamA_PAsqualo_R19b/controller1/transect controller/yaw_controller/Yaw PID controller/compute_velocity_error ==
  data: enable input; err_vel output; v_des input; est_meas input
function err_vel = fcn(enable,v_des,est_meas)
if enable == 1
   err_vel =  v_des - est_meas(12);
else
    err_vel = 0;
end
end

== matlab function TeamA_PAsqualo_R19b/controller1/turning controller/heave_controller/Heave PID controller/compute_position_errors ==
  data: enable input; err_pos output; ref input; est_state input; areaOfInterestCorner parameter
function err_pos = fcn(enable, ref, est_state,areaOfInterestCorner)
references_NED = zeros(3,1);
est_state_NED  = zeros(3,1);
phi = est_state(4);
th  = est_state(5);
psi = est_state(6);
coder.extrinsic('evalin','wgs84Ellipsoid','geodetic2ned');
orig = [areaOfInterestCorner(1)   areaOfInterestCorner(2)   areaOfInterestCorner(3)]'; %origine terna NED
wgs84 = wgs84Ellipsoid;
if enable == 1
   % Cambiamento di riferimento da WGS84 a NED frame
   [x_ref, y_ref, z_ref] = geodetic2ned(ref(1),ref(2),ref(3),orig(1),orig(2),orig(3),wgs84);
   references_NED = [x_ref, y_ref, z_ref]';
   [x_est, y_est, z_est] = geodetic2ned(est_state(1),est_state(2),est_state(3),orig(1),orig(2),orig(3),wgs84);
   est_state_NED  =  [x_est, y_est, z_est]';
   est_state_NED = [est_state_NED(1);est_state_NED(2);est_state(3)];
   % Calcolo errore posizione da NED a BODY frame
   err_NED  = references_NED - est_state_NED;
   R_z_psi = [cos(psi)    sin(psi)     0;
              -sin(psi)   cos(psi)     0;
                 0           0         1];
          
   R_y_th =  [cos(th)        0      -sin(th);
                 0           1         0;
              sin(th)        0       cos(th)];
       
   R_x_phi = [   1           0             0;
                 0         cos(phi)    sin(phi);
                 0        -sin(phi)    cos(phi)];
          
   R_NB = ((R_z_psi')*(R_y_th')*(R_x_phi'))';
   err_pos_BODY = R_NB * err_NED;
   err_pos = err_pos_BODY(3);
else
   err_pos = 0;
end
end

== matlab function TeamA_PAsqualo_R19b/controller1/turning controller/heave_controller/Heave PID controller/compute_velocity_error ==
  data: enable input; err_vel output; v_des input; est_meas input
function err_vel = fcn(enable,v_des,est_meas)
if enable == 1
   err_vel =  v_des - est_meas(9);
else
    err_vel = 0;
end
end

== matlab function TeamA_PAsqualo_R19b/controller1/turning controller/pitch_controller/Pitch PID controller/compute_orientation_errors ==
  data: enable input; err_orient output; ref input; est_state input
function err_orient = fcn(enable, ref, est_state)
coder.extrinsic('wrapToPi');
err_orient = 0;
phi = est_state(4);
th  = est_state(5);
%
J_inv = [1       0          -sin(th); 
         0   cos(phi)  cos(th)*sin(phi);
         0  -sin(phi)  cos(th)*cos(phi)];
if enable == 1
   err_orient_1 = wrapToPi(J_inv*([ref(4);ref(5);ref(6)] -...
                           [est_state(4);est_state(5);est_state(6)]));
else 
   err_orient_1 = zeros(3,1);
end
err_orient = err_orient_1(2);
end

== matlab function TeamA_PAsqualo_R19b/controller1/turning controller/pitch_controller/Pitch PID controller/compute_velocity_error ==
  data: enable input; err_vel output; v_des input; est_meas input
function err_vel = fcn(enable,v_des,est_meas)
if enable == 1
   err_vel =  v_des - est_meas(11);
else
    err_vel = 0;
end
end

== matlab function TeamA_PAsqualo_R19b/controller1/turning controller/roll_controller/Roll PID controller/compute_orientation_errors ==
  data: enable input; err_orient output; ref input; est_state input
function err_orient = fcn(enable, ref, est_state)
coder.extrinsic('wrapToPi');
err_orient = 0;
phi = est_state(4);
th  = est_state(5);
%
J_inv = [1       0          -sin(th); 
         0   cos(phi)  cos(th)*sin(phi);
         0  -sin(phi)  cos(th)*cos(phi)];
if enable == 1
   err_orient_1 = wrapToPi(J_inv*([ref(4);ref(5);ref(6)] -...
                           [est_state(4);est_state(5);est_state(6)]));
else 
   err_orient_1 = zeros(3,1);
end
err_orient = err_orient_1(1);
end

== matlab function TeamA_PAsqualo_R19b/controller1/turning controller/roll_controller/Roll PID controller/compute_velocity_error ==
  data: enable input; err_vel output; v_des input; est_meas input
function err_vel = fcn(enable,v_des,est_meas)
if enable == 1
   err_vel =  v_des - est_meas(10);
else
    err_vel = 0;
end
end

== matlab function TeamA_PAsqualo_R19b/controller1/turning controller/surge_controller/Surge PID controller/ compute_velocity_error ==
  data: enable input; ref input; est_meas input; err_vel output
function err_vel = fcn(enable, ref, est_meas)
if  enable == 1
    err_vel = ref(7) - est_meas(7);
else
    err_vel = 0;
end
end

== matlab function TeamA_PAsqualo_R19b/controller1/turning controller/sway_controller/Sway PID controller/compute_position_errors ==
  data: enable input; err_pos output; ref input; est_state input; areaOfInterestCorner parameter
function err_pos = fcn(enable, ref, est_state,areaOfInterestCorner)
references_NED = zeros(3,1);
est_state_NED  = zeros(3,1);
phi = est_state(4);
th  = est_state(5);
psi = est_state(6);
coder.extrinsic('evalin','wgs84Ellipsoid','geodetic2ned'); 
orig = [areaOfInterestCorner(1)   areaOfInterestCorner(2)   areaOfInterestCorner(3)]'; %origine terna NED
wgs84 = wgs84Ellipsoid;
if enable == 1
    % Cambiamento di riferimento da WGS84 a NED frame
   [x_ref, y_ref, z_ref] = geodetic2ned(ref(1),ref(2),ref(3),orig(1),orig(2),orig(3),wgs84);
   references_NED = [x_ref, y_ref, z_ref]';
   [x_est, y_est, z_est] = geodetic2ned(est_state(1),est_state(2),est_state(3),orig(1),orig(2),orig(3),wgs84);
   est_state_NED  =  [x_est, y_est, est_state(3)]';
   % Calcolo errore posizione da NED a BODY frame, con componente east
   err_NED  = references_NED - est_state_NED;
   R_z_psi = [cos(psi)    sin(psi)     0;
              -sin(psi)   cos(psi)     0;
                 0           0         1];
          
   R_y_th =  [cos(th)        0      -sin(th);
                 0           1         0;
              sin(th)        0       cos(th)];
       
   R_x_phi = [   1           0             0;
                 0         cos(phi)    sin(phi);
                 0        -sin(phi)    cos(phi)];
          
   R_NB = ((R_z_psi')*(R_y_th')*(R_x_phi'))';
   err_pos_BODY = R_NB * err_NED;
   err_pos = err_pos_BODY(2);
else
   err_pos = 0;
end
end

== matlab function TeamA_PAsqualo_R19b/controller1/turning controller/sway_controller/Sway PID controller/compute_velocity_error ==
  data: enable input; err_vel output; v_des input; est_meas input
function err_vel = fcn(enable,v_des,est_meas)
if enable == 1
   err_vel =  v_des - est_meas(8);
else
    err_vel = 0;
end
end

== matlab function TeamA_PAsqualo_R19b/controller1/turning controller/yaw_controller/Yaw PID controller/compute_orientation_errors ==
  data: enable input; err_orient output; ref input; est_state input
function err_orient = fcn(enable, ref, est_state)
coder.extrinsic('wrapToPi');
err_orient = 0;
phi = est_state(4);
th  = est_state(5);
%
J_inv = [1       0          -sin(th); 
         0   cos(phi)  cos(th)*sin(phi);
         0  -sin(phi)  cos(th)*cos(phi)];
if enable == 1
   err_orient_1 = wrapToPi(J_inv*([ref(4);ref(5);ref(6)] -...
                           [est_state(4);est_state(5);est_state(6)]));
else 
   err_orient_1 = zeros(3,1);
end
err_orient = err_orient_1(3);
end

== matlab function TeamA_PAsqualo_R19b/controller1/turning controller/yaw_controller/Yaw PID controller/compute_velocity_error ==
  data: enable input; err_vel output; v_des input; est_meas input
function err_vel = fcn(enable,v_des,est_meas)
if enable == 1
   err_vel =  v_des - est_meas(12);
else
    err_vel = 0;
end
end

== matlab function TeamA_PAsqualo_R19b/Navigazione/MATLAB Function ==
  data: u input size=[3,1]; y output
function y = fcn(u)

if norm(u) > 1e5
	y = 0;
else
	y = 1;
end

end
